simulink model "DDC"  (R2021b)
settings: Solver=FixedStepDiscrete  StartTime=0.0  StopTime=4  FixedStep=1/69.333e3  RelTol=1e-3
PreLoadFcn:
  | gsmcoeffs
libraries: dspmlti4 x5, dspobslib x1, dspsrcs4 x1, dspmathops x1
settings Model: Creator=denis  LastModifiedBy=denis
settings SolverCC: AlgebraicLoopSolver=TrustRegion
settings DataIOCC: LimitDataPoints=on  SaveFormat=Array  ReturnWorkspaceOutputs=off
settings OptimizationCC: LifeSpan=inf
settings DebuggingCC: SolverPrmCheckMsg=warning  SFUnexpectedBacktrackingDiag=warning  SFNoUnconditionalDefaultTransitionDiag=warning  SFExecutionAtInitializationDiag=none  SFMachineParentedDataDiag=warning  ArithmeticOperatorsInVariantConditions=warning
settings HardwareCC: ProdBitPerPointer=32  ProdBitPerSizeT=32  ProdBitPerPtrDiffT=32  ProdLargestAtomicFloat=None  ProdIntDivRoundTo=Undefined  ProdEndianess=Unspecified  ProdWordSize=32  ProdHWDeviceType=32-bit Generic
settings ModelReferenceCC: PropagateSignalLabelsOutOfModel=off
settings SFSimCC: SimUseLocalCustomCode=off  CustomCodeUndefinedFunction=UseInterfaceOnly
settings RTWCC: RTWUseLocalCustomCode=off
settings CodeAppCC: StateflowObjectComments=on
settings GRTTargetCC: TargetLangStandard=C89/C90 (ANSI)
settings ConfigComp: CovMetricSettings=dw  CovSaveCumulativeToWorkspaceVar=on  CovSaveSingleToWorkspaceVar=on  CovExternalEMLEnable=off

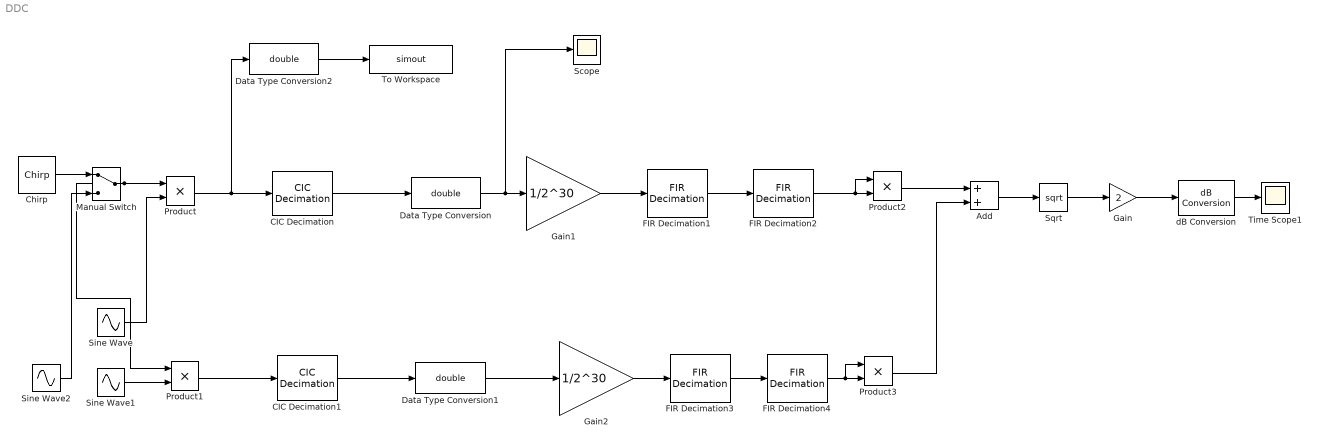
== system DDC ==
  Add : Sum
  CIC Decimation : dspobslib/CIC Decimation  filtFrom=Dialog  filtobj=Hm_decim  ftype=Decimator  R=64  M=1  N=5  filterInternals=Full precision  BPS=[16 16 16 16]  FLPS=0  outputWordLength=20  outputFracLength=0  launchFVT=off  framing=Maintain input frame rate  RateOptions=Allow multirate processing
      settings: SourceProductBaseCode=DS
  CIC Decimation1 : dspmlti4/CIC Decimation  filtFrom=Dialog parameters  filtobj=Hm_decim  ftype=Decimator  R=64  M=1  N=5  filterInternals=Full precision  BPS=[16 16 16 16]  FLPS=0  outputWordLength=20  outputFracLength=0  launchFVT=off  framing=Maintain input frame rate  RateOptions=Allow multirate processing
      settings: SourceProductBaseCode=DS
  Chirp : dspsrcs4/Chirp  sweep=Linear  mode=Unidirectional  f0=10000  f1=20000  t1=4  Tsweep=4  phase=0  Ts=1/69.333e3  spf=1  datatype=Double  OutputFrames=on
  Data Type Conversion : DataTypeConversion  OutDataTypeStr=double
  Data Type Conversion1 : DataTypeConversion  OutDataTypeStr=double
  Data Type Conversion2 : DataTypeConversion  OutDataTypeStr=double
  FIR Decimation1 : dspmlti4/FIR Decimation  FilterSource=Dialog parameters  h=cfir  D=2  filtStruct=Direct form  FilterObject=Hm_firdecim  InputProcessing=Columns as channels (frame based)  framing=Allow multirate processing  inputOffset=0  outputBufInitCond=0  roundingMode=Floor  overflowMode=off  firstCoeffDataTypeStr=Inherit: Same word length as input  firstCoeffMin=[]  firstCoeffMax=16  firstCoeffLastDataTypeStr=Inherit: Same word length as input  outputMode=Binary point scaling  outputWordLength=20  outputFracLength=12  outputDataTypeStr=fixdt(1,20,12)  outputMin=[]  outputMax=[]  outputLastDataTypeStr=fixdt(1,20,12)
  FIR Decimation2 : dspmlti4/FIR Decimation  FilterSource=Dialog parameters  h=pfir  D=2  filtStruct=Direct form  FilterObject=Hm_firdecim  InputProcessing=Columns as channels (frame based)  framing=Allow multirate processing  inputOffset=0  outputBufInitCond=0  roundingMode=Floor  overflowMode=off  firstCoeffDataTypeStr=Inherit: Same word length as input  firstCoeffMin=[]  firstCoeffMax=16  firstCoeffLastDataTypeStr=Inherit: Same word length as input  outputMode=Binary point scaling  outputWordLength=20  outputFracLength=12  outputDataTypeStr=fixdt(1,20,12)  outputMin=[]  outputMax=[]  outputLastDataTypeStr=fixdt(1,20,12)
  FIR Decimation3 : dspmlti4/FIR Decimation  FilterSource=Dialog parameters  h=cfir  D=2  filtStruct=Direct form  FilterObject=Hm_firdecim  InputProcessing=Columns as channels (frame based)  framing=Allow multirate processing  inputOffset=0  outputBufInitCond=0  roundingMode=Floor  overflowMode=off  firstCoeffDataTypeStr=Inherit: Same word length as input  firstCoeffMin=[]  firstCoeffMax=16  firstCoeffLastDataTypeStr=Inherit: Same word length as input  outputMode=Binary point scaling  outputWordLength=20  outputFracLength=12  outputDataTypeStr=fixdt(1,20,12)  outputMin=[]  outputMax=[]  outputLastDataTypeStr=fixdt(1,20,12)
  FIR Decimation4 : dspmlti4/FIR Decimation  FilterSource=Dialog parameters  h=pfir  D=2  filtStruct=Direct form  FilterObject=Hm_firdecim  InputProcessing=Columns as channels (frame based)  framing=Allow multirate processing  inputOffset=0  outputBufInitCond=0  roundingMode=Floor  overflowMode=off  firstCoeffDataTypeStr=Inherit: Same word length as input  firstCoeffMin=[]  firstCoeffMax=16  firstCoeffLastDataTypeStr=Inherit: Same word length as input  outputMode=Binary point scaling  outputWordLength=20  outputFracLength=12  outputDataTypeStr=fixdt(1,20,12)  outputMin=[]  outputMax=[]  outputLastDataTypeStr=fixdt(1,20,12)
  Gain : Gain  Gain=2
  Gain1 : Gain  Gain=1/2^30
  Gain2 : Gain  Gain=1/2^30
  Manual Switch : ManualSwitch
  Product : Product  OutMin=0  OutMax=1  OutDataTypeStr=fixdt(1,16,14)
  Product1 : Product  OutMin=0  OutMax=1  OutDataTypeStr=fixdt(1,16,14)
  Product2 : Product  OutMin=0  OutMax=1  OutDataTypeStr=double
  Product3 : Product  OutMin=0  OutMax=1  OutDataTypeStr=double
  Scope : Scope
  Sine Wave : Sin  Frequency=14.44e3*2*pi  SampleTime=1/69.333e3
  Sine Wave1 : Sin  Frequency=14.44e3*2*pi  Phase=pi/2  SampleTime=1/69.333e3
  Sine Wave2 : Sin  Frequency=14.44e3*2*pi  Phase=pi/2  SampleTime=1/69.333e3
  Sqrt : Sqrt  SaturateOnIntegerOverflow=on
  Time Scope1 : Scope
  To Workspace : ToWorkspace  VariableName=simout  SampleTime=-1
      settings: Save2DSignal=2-D array (concatenate along first dimension)
  dB Conversion : dspmathops/dB Conversion  dBtype=dB  intype=Amplitude  R=1  fuzz=on
  wires:
  Sine Wave2/1 -> Manual Switch/2
  Chirp/1 -> Manual Switch/1
  dB Conversion/1 -> Time Scope1/1
  Gain2/1 -> FIR Decimation3/1
  Gain1/1 -> FIR Decimation1/1
  Gain/1 -> dB Conversion/1
  Sqrt/1 -> Gain/1
  Add/1 -> Sqrt/1
  Product3/1 -> Add/2
  Product2/1 -> Add/1
  Data Type Conversion1/1 -> Gain2/1
  FIR Decimation3/1 -> FIR Decimation4/1
  Sine Wave1/1 -> Product1/2
  Data Type Conversion/1 -> Scope/1, Gain1/1
  FIR Decimation1/1 -> FIR Decimation2/1
  Product/1 -> Data Type Conversion2/1, CIC Decimation/1
  CIC Decimation/1 -> Data Type Conversion/1
  Sine Wave/1 -> Product/2
  Manual Switch/1 -> Product/1, Product1/1
  FIR Decimation4/1 -> Product3/1, Product3/2
  Product1/1 -> CIC Decimation1/1
  CIC Decimation1/1 -> Data Type Conversion1/1
  FIR Decimation2/1 -> Product2/1, Product2/2
  Data Type Conversion2/1 -> To Workspace/1
